simulink model "Q4_Ball_Beam_slx"  (R2018b)
settings: Solver=ode45  StartTime=0.0  StopTime=20  MaxStep=0.01  RelTol=1e-3  EnableMultiTasking=on
undefined symbols (not defined in the file): c, d, g, Kd1, Kd2, Kd3, Kd4, Ki1, Ki2, Ki3, Ki4, Kp1, Kp2, Kp3, Kp4, L, m, nG, nSat, nVR, T1, T2, T3, T4
libraries: checkpacklib x4, slctrlblks x1
settings Model: Creator=Home  LastModifiedBy=Erfan Etesami
settings DataIOCC: LimitDataPoints=on
settings OptimizationCC: LifeSpan=inf
settings DebuggingCC: SFUnexpectedBacktrackingDiag=warning  SFNoUnconditionalDefaultTransitionDiag=warning  SFExecutionAtInitializationDiag=none
settings HardwareCC: ProdBitPerSizeT=32  ProdBitPerPtrDiffT=32  ProdWordSize=32  ProdHWDeviceType=Specified
settings SFSimCC: SimUseLocalCustomCode=off
settings RTWCC: RTWUseLocalCustomCode=off
settings CodeAppCC: StateflowObjectComments=on
settings GRTTargetCC: TargetLangStandard=C89/C90 (ANSI)  GeneratePreprocessorConditionals=Disable all
settings ConfigComp: CovMetricSettings=dw  CovHtmlReporting=on  CovSaveCumulativeToWorkspaceVar=on  CovSaveSingleToWorkspaceVar=on  CovExternalEMLEnable=off  CovSFcnEnable=off
settings SimscapeCC: SimscapeNominalValues="[{\"value\":\"10\",\"unit\":\"V\"},{\"value\":\"1\",\"unit\":\"A\"},{\"value\":\"10\",\"unit\":\"N*m\"},{\"value\":\"10\",\"unit\":\"bar\"},{\"value\":\"100\",\"unit\":\"kJ/kg\"},{\"value\":\"1\",\"unit\":\"kW\"},{\"value\":\"300\",\"unit\":\"K\"},{\"value\":\"100\",\"unit\":\"cm^3/s\"},{\"value\":\"1\",\"unit\":\"kN\"},{\"value\":\"1\",\"unit\":\"g/cm^3\"},{\"value\":\"1\",\"unit\":\"l\"},{\"value\":\"1\",\"unit\":\"cm^2\"},{\"value\":\"60\",\"unit\":\"Hz\"}]"  SimscapeLogType=all  SimscapeLogDataHistory=10000

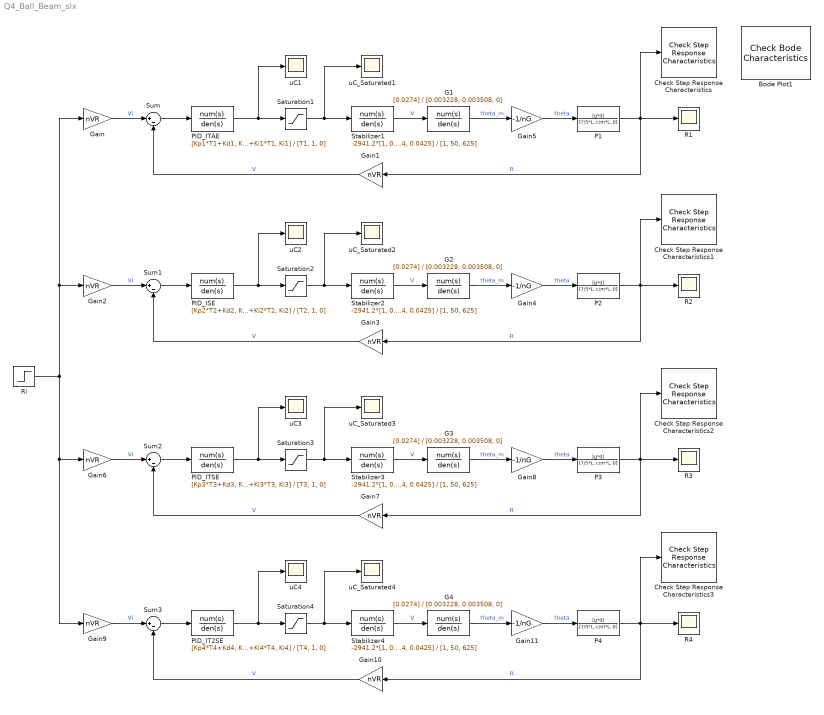
== system Q4_Ball_Beam_slx ==
  " PID_ISE" : TransferFcn  Numerator=[Kp2*T2+Kd2, Kp2+Ki2*T2, Ki2]  Denominator=[T2, 1, 0]
  " PID_IT2SE" : TransferFcn  Numerator=[Kp4*T4+Kd4, Kp4+Ki4*T4, Ki4]  Denominator=[T4, 1, 0]
  " PID_ITAE" : TransferFcn  Numerator=[Kp1*T1+Kd1, Kp1+Ki1*T1, Ki1]  Denominator=[T1, 1, 0]
  " PID_ITSE" : TransferFcn  Numerator=[Kp3*T3+Kd3, Kp3+Ki3*T3, Ki3]  Denominator=[T3, 1, 0]
  Bode Plot1 : slctrlblks/Model Verification/Check Bode  Characteristics  InstantiateOnLoad=on  SaveOperatingPoints=off  LinearizationIOs={'/Ri ', 1, 'in', 'on', '';'/P1', 1, 'out', 'on', ''}  LinearizeAt=SnapshotTimes  SnapshotTimes=[0]  TriggerType=rising  SampleTime=auto  RateConversionMethod=zoh  PreWarpFreq=10  UseExactDelayModel=off  UseFullBlockNameLabels=off  UseBusSignalLabels=off  enabled=on  stopWhenAssertionFail=off  export=off  ViewDlgPos=[411.4 133.8 568 461.6]  OpenViewOnLoad=on  LaunchViewOnOpen=on  FrequencyUnits=rad/s  MagnitudeUnits=dB  PhaseUnits=deg  TimeUnits=seconds  EnableUpperBound=off  UpperBoundFrequencies=[]  UpperBoundMagnitudes=[]  EnableLowerBound=off  LowerBoundFrequencies=[]  LowerBoundMagnitudes=[]
      settings: SourceProductName=Simulink Control Design
  Check Step Response Characteristics{,1..3} (4 alike) : checkpacklib/Check Step Response  Characteristics  InstantiateOnLoad=on  enabled=on  stopWhenAssertionFail=on  export=off  ViewDlgPos=[241 204.2 509.6 389.6]  OpenViewOnLoad=off  LaunchViewOnOpen=on  TimeUnits=seconds  EnableStepResponseBound=on  InitialValue=0  FinalValue=L/2  StepTime=0  RiseTime=5  PercentRise=80  SettlingTime=6  PercentSettling=2  PercentOvershoot=20  PercentUndershoot=1
  "G1 " : TransferFcn  Numerator=[0.0274]  Denominator=[0.003228, 0.003508, 0]
  G2 : TransferFcn  Numerator=[0.0274]  Denominator=[0.003228, 0.003508, 0]
  G3 : TransferFcn  Numerator=[0.0274]  Denominator=[0.003228, 0.003508, 0]
  G4 : TransferFcn  Numerator=[0.0274]  Denominator=[0.003228, 0.003508, 0]
  Gain{,1..3,6..7,9..10} (8 alike) : Gain  Gain=nVR
  Gain{4..5,8,11} (4 alike) : Gain  Gain=-1/nG
  P{1..4} (4 alike) : TransferFcn  Numerator=[g*d]  Denominator=[7/5*L, c/m*L, 0]
  R{1..4} (4 alike) : Scope
  "Ri " : Step  Time=0  After=L/2  SampleTime=0
  "Saturation1 " : Saturate  UpperLimit=nSat  LowerLimit=-nSat
  "Saturation2 " : Saturate  UpperLimit=nSat  LowerLimit=-nSat
  "Saturation3 " : Saturate  UpperLimit=nSat  LowerLimit=-nSat
  "Saturation4 " : Saturate  UpperLimit=nSat  LowerLimit=-nSat
  Stabilizer{1..4} (4 alike) : TransferFcn  Numerator=-2941.2*[1, 0.4, 0.0425]  Denominator=[1, 50, 625]
  Sum{,1..3} (4 alike) : Sum  Inputs=|+-
  "uC1 " : Scope
  uC2 : Scope
  uC3 : Scope
  uC4 : Scope
  "uC_Saturated1 " : Scope
  uC_Saturated2 : Scope
  uC_Saturated3 : Scope
  uC_Saturated4 : Scope
  wires:
  Gain/1 -> Sum/1  "Vi"
  Sum/1 -> " PID_ITAE"/1
  "G1 "/1 -> Gain5/1  "theta_m"
  Gain1/1 -> Sum/2  "V"
  P1/1 -> R1/1, Gain1/1, Check Step Response Characteristics/1  "R"
  Gain5/1 -> P1/1  "theta"
  Stabilizer1/1 -> "G1 "/1  "V"
  " PID_ITAE"/1 -> "Saturation1 "/1, "uC1 "/1
  "Saturation1 "/1 -> Stabilizer1/1, "uC_Saturated1 "/1
  "Saturation2 "/1 -> uC_Saturated2/1, Stabilizer2/1
  " PID_ISE"/1 -> uC2/1, "Saturation2 "/1
  Stabilizer2/1 -> G2/1  "V"
  Gain4/1 -> P2/1  "theta"
  P2/1 -> R2/1, Gain3/1, Check Step Response Characteristics1/1  "R"
  Gain3/1 -> Sum1/2  "V"
  G2/1 -> Gain4/1  "theta_m"
  Sum1/1 -> " PID_ISE"/1
  Gain2/1 -> Sum1/1  "Vi"
  Gain6/1 -> Sum2/1  "Vi"
  Sum2/1 -> " PID_ITSE"/1
  G3/1 -> Gain8/1  "theta_m"
  Gain7/1 -> Sum2/2  "V"
  P3/1 -> Check Step Response Characteristics2/1, R3/1, Gain7/1  "R"
  Gain8/1 -> P3/1  "theta"
  Stabilizer3/1 -> G3/1  "V"
  " PID_ITSE"/1 -> "Saturation3 "/1, uC3/1
  "Saturation3 "/1 -> Stabilizer3/1, uC_Saturated3/1
  "Ri "/1 -> Gain6/1, Gain9/1, Gain2/1, Gain/1
  "Saturation4 "/1 -> uC_Saturated4/1, Stabilizer4/1
  " PID_IT2SE"/1 -> uC4/1, "Saturation4 "/1
  Stabilizer4/1 -> G4/1  "V"
  Gain11/1 -> P4/1  "theta"
  P4/1 -> Gain10/1, R4/1, Check Step Response Characteristics3/1  "R"
  Gain10/1 -> Sum3/2  "V"
  G4/1 -> Gain11/1  "theta_m"
  Sum3/1 -> " PID_IT2SE"/1
  Gain9/1 -> Sum3/1  "Vi"
